simulink model "blocks"  (R2019a)
settings: Solver=VariableStepAuto  StartTime=0.0  StopTime=10.0  RelTol=1e-3
settings Model: Creator=adeye  LastModifiedBy=adeye

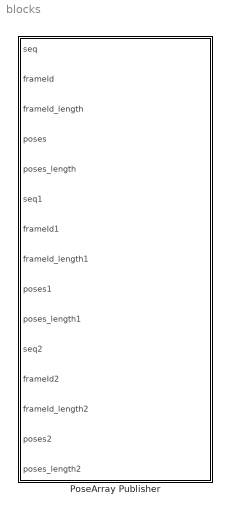
== system blocks ==
  PoseArray Publisher : Subsystem  mask{topic='/pose_otherCar', message_type='geometry_msgs/PoseArray', port=9090, timeout=2}
      mask prompts: topic "Topic name"; message_type "Message type"; timeout "Timeout (s)"

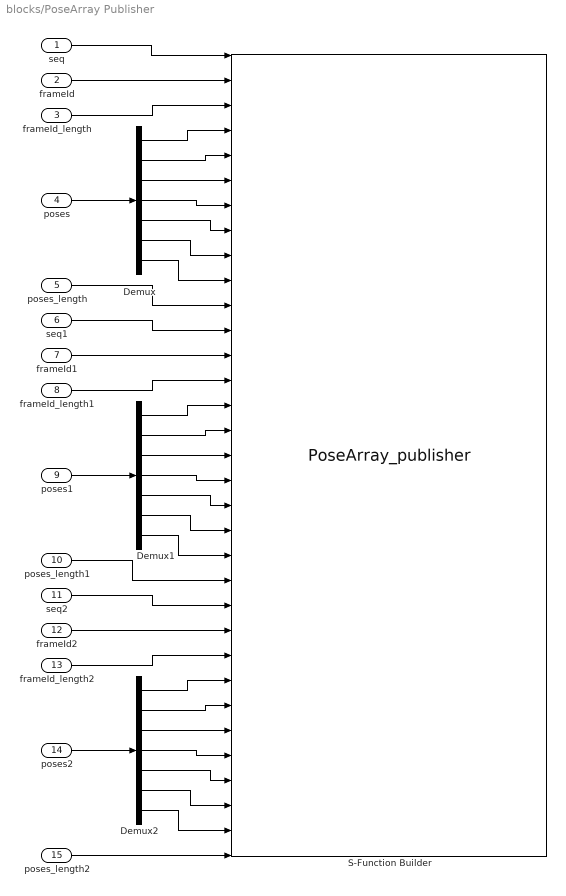
== system blocks/PoseArray Publisher ==
  seq : Inport
  frameId : Inport  Port=2
  frameId_length : Inport  Port=3
  poses : Inport  Port=4
  poses_length : Inport  Port=5
  seq1 : Inport  Port=6
  frameId1 : Inport  Port=7
  frameId_length1 : Inport  Port=8
  poses1 : Inport  Port=9
  poses_length1 : Inport  Port=10
  seq2 : Inport  Port=11
  frameId2 : Inport  Port=12
  frameId_length2 : Inport  Port=13
  poses2 : Inport  Port=14
  poses_length2 : Inport  Port=15
  Demux : Demux  Outputs=7
  Demux1 : Demux  Outputs=7
  Demux2 : Demux  Outputs=7
  S-Function Builder : S-Function  InitFcn=try, set_param(gcb,'FunctionName','PoseArray_publisher'), end  FunctionName=PoseArray_publisher  Parameters=int8(topic),int8(message_type),port,timeout  SFunctionModules=PoseArray_publisher_wrapper rosbridge_functions  SFunctionDeploymentMode=off  EnableBusSupport=off  mask(S-Function Builder){}
      mask help: Simulink:masks:SFunctionBuilder_MD
      mask init:
      | val = [[.9  0.75 0.75 1 1 .9 .9 1]',[1 1 0.75 0.75 .9 .9 1 .9]'];try , sys = get_param(gcb,'SfunBuilderFcnName');if isempty(sys), sys = get_param(gcb,'FunctionName'); end,catch, sys = get_param(gcb,'FunctionName'); end
      settings: CopyFcn=set_param(gcbh,'LinkStatus','none')  PreSaveFcn=try, set_param(gcb,'FunctionName','PoseArray_publisher'), end  OpenFcn=sfunctionwizard(gcbh)
      mask Display: plot(val(:,1),val(:,2)),disp(sys), port_label('input',1,'seq'), port_label('input',2,'frameId'), port_label('input',3,'frameId_length'), port_label('input',4,'positionX'), port_label('input',5,'positionY'), port_label('input',6,'positionZ'), port_label('input',7,'orientationW'), port_label('input',8,'orientationX'), port_label('input',9,'orientationY'), port_label('input',10,'orientationZ'), port_label('input',11,'poses_length'), port_label('input',12,'seq1'), port_label('input',13,'frameId1'), port_label('input',14,'frameId_length1'), port_label('input',15,'positionX1'), port_label('input',16,'positionY1'), port_label('input',17,'positionZ1'), port_label('input',18,'orientationW1'), port_label('input',19,'orientationX1'), port_label('input',20,'orientationY1'), port_label('input',21,'orientationZ1'), port_label('input',22,'poses_length1'), port_label('input',23,'seq2'), port_label('input',24,'frameId2'), port_label('input',25,'frameId_length2'), port_label('input',26,'positionX2'), port_label('input',27,'positionY2'), port_label('input',28,'positionZ2'), port_label('input',29,'orientationW2'), port_label('input',30,'orientationX2'), port_label('input',31,'orientationY2'), port_label('input',32,'orientationZ2'), port_label('input',33,'poses_length2')
  wires:
  seq/1 -> S-Function Builder/1
  Demux/1 -> S-Function Builder/4
  Demux/2 -> S-Function Builder/5
  Demux/3 -> S-Function Builder/6
  Demux/4 -> S-Function Builder/7
  Demux/5 -> S-Function Builder/8
  Demux/6 -> S-Function Builder/9
  Demux/7 -> S-Function Builder/10
  frameId_length/1 -> S-Function Builder/3
  frameId/1 -> S-Function Builder/2
  poses/1 -> Demux/1
  poses_length/1 -> S-Function Builder/11
  frameId1/1 -> S-Function Builder/13
  frameId_length1/1 -> S-Function Builder/14
  seq1/1 -> S-Function Builder/12
  Demux1/6 -> S-Function Builder/20
  Demux1/2 -> S-Function Builder/16
  Demux1/7 -> S-Function Builder/21
  Demux1/5 -> S-Function Builder/19
  Demux1/3 -> S-Function Builder/17
  Demux1/4 -> S-Function Builder/18
  Demux1/1 -> S-Function Builder/15
  poses1/1 -> Demux1/1
  poses_length1/1 -> S-Function Builder/22
  seq2/1 -> S-Function Builder/23
  frameId2/1 -> S-Function Builder/24
  frameId_length2/1 -> S-Function Builder/25
  Demux2/6 -> S-Function Builder/31
  Demux2/4 -> S-Function Builder/29
  Demux2/3 -> S-Function Builder/28
  Demux2/2 -> S-Function Builder/27
  Demux2/7 -> S-Function Builder/32
  poses2/1 -> Demux2/1
  Demux2/1 -> S-Function Builder/26
  Demux2/5 -> S-Function Builder/30
  poses_length2/1 -> S-Function Builder/33
